simulink library "wabha_method"  (R2021b)
settings: Solver=VariableStepAuto  StartTime=0.0  StopTime=10.0  RelTol=1e-3
libraries: sharedutil x2, mat_3x3 x1
settings Model: Creator=white  LastModifiedBy=white

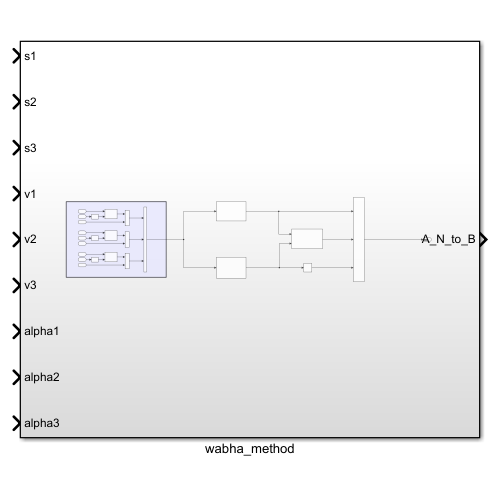
[thumbnail: Simulink's stored preview of the top-level diagram]
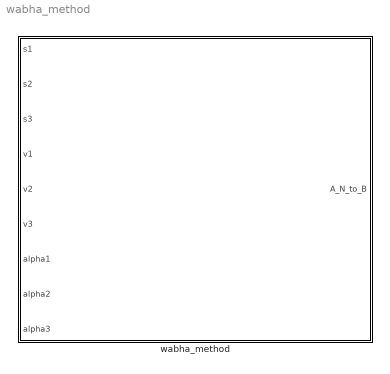
== system wabha_method ==
  wabha_method : Subsystem

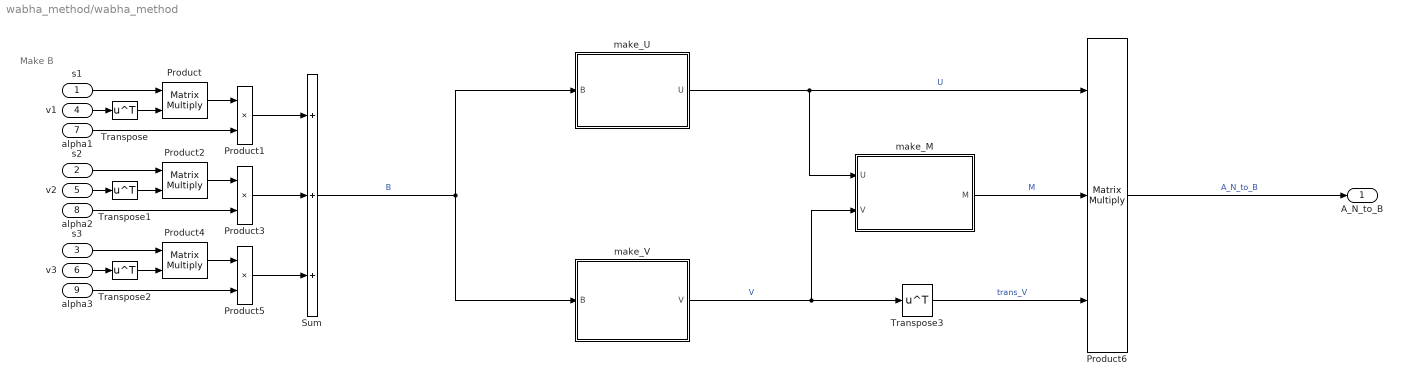
== system wabha_method/wabha_method ==
  note: Make B
  s1 : Inport
  s2 : Inport  Port=2
  s3 : Inport  Port=3
  v1 : Inport  Port=4
  v2 : Inport  Port=5
  v3 : Inport  Port=6
  alpha1 : Inport  Port=7
  alpha2 : Inport  Port=8
  alpha3 : Inport  Port=9
  Product : Product  Multiplication=Matrix(*)
  Product1 : Product
  Product2 : Product  Multiplication=Matrix(*)
  Product3 : Product
  Product4 : Product  Multiplication=Matrix(*)
  Product5 : Product
  Product6 : Product  Inputs=3  Multiplication=Matrix(*)
  Sum : Sum  Inputs=+++
  Transpose{,1..3} (4 alike) : Math  Operator=transpose  SaturateOnIntegerOverflow=on
  make_M : Subsystem
  make_U : Subsystem
  make_V : Subsystem
  A_N_to_B : Outport
  wires:
  v1/1 -> Transpose/1
  Transpose/1 -> Product/2
  s1/1 -> Product/1
  alpha1/1 -> Product1/2
  Product/1 -> Product1/1
  Product1/1 -> Sum/1
  Product2/1 -> Product3/1
  alpha2/1 -> Product3/2
  s2/1 -> Product2/1
  Transpose1/1 -> Product2/2
  v2/1 -> Transpose1/1
  Product3/1 -> Sum/2
  Product5/1 -> Sum/3
  v3/1 -> Transpose2/1
  Transpose2/1 -> Product4/2
  s3/1 -> Product4/1
  alpha3/1 -> Product5/2
  Product4/1 -> Product5/1
  Sum/1 -> make_V/1(B), make_U/1(B)  "B"
  make_U/1(U) -> make_M/1(U), Product6/1  "U"
  make_V/1(V) -> make_M/2(V), Transpose3/1  "V"
  Transpose3/1 -> Product6/3  "trans_V"
  make_M/1(M) -> Product6/2  "M"
  Product6/1 -> A_N_to_B/1  "A_N_to_B"

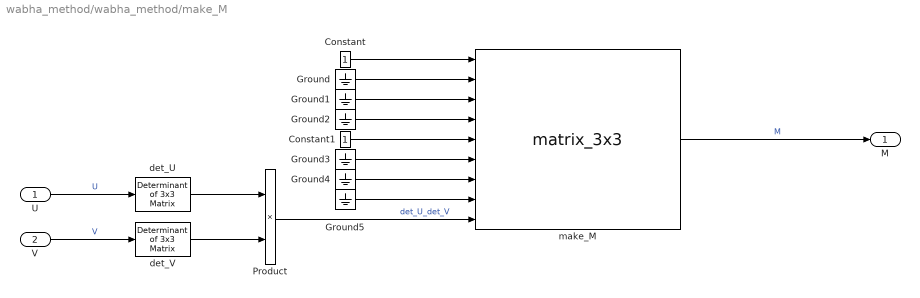
== system wabha_method/wabha_method/make_M ==
  U : Inport
  V : Inport  Port=2
  Constant : Constant
  Constant1 : Constant
  Ground{,1..5} (6 alike) : Ground
  Product : Product
  det_U : sharedutil/Determinant of 3x3 Matrix  aMode=aMode
      settings: SourceProductBaseCode=AE,PW,DR,MT,UV,VE
  det_V : sharedutil/Determinant of 3x3 Matrix  aMode=aMode
      settings: SourceProductBaseCode=AE,PW,DR,MT,UV,VE
  make_M : mat_3x3/matrix_3x3  SystemSampleTime=-1  VariantActivationTime=update diagram  Latency=0  AutoFrameSizeCalculation=off
  M : Outport
  wires:
  V/1 -> det_V/1  "V"
  U/1 -> det_U/1  "U"
  make_M/1 -> M/1  "M"
  Constant/1 -> make_M/1
  Ground/1 -> make_M/2
  Ground1/1 -> make_M/3
  Ground2/1 -> make_M/4
  Ground3/1 -> make_M/6
  Ground4/1 -> make_M/7
  Ground5/1 -> make_M/8
  Constant1/1 -> make_M/5
  det_V/1 -> Product/2
  det_U/1 -> Product/1
  Product/1 -> make_M/9  "det_U_det_V"

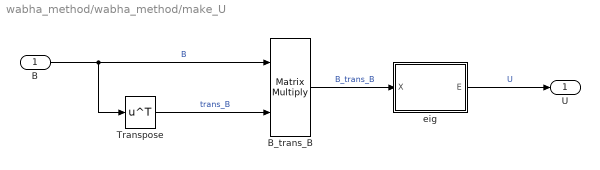
== system wabha_method/wabha_method/make_U ==
  B : Inport
  B_trans_B : Product  Multiplication=Matrix(*)
  Transpose : Math  Operator=transpose  SaturateOnIntegerOverflow=on
  eig : MATLAB Function  TreatAsAtomicUnit=on
  U : Outport
  wires:
  B/1 -> B_trans_B/1, Transpose/1  "B"
  Transpose/1 -> B_trans_B/2  "trans_B"
  B_trans_B/1 -> eig/1(X)  "B_trans_B"
  eig/1(E) -> U/1  "U"

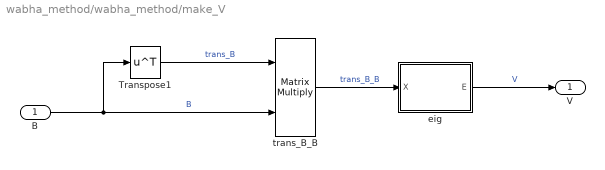
== system wabha_method/wabha_method/make_V ==
  B : Inport
  Transpose1 : Math  Operator=transpose  SaturateOnIntegerOverflow=on
  eig : MATLAB Function  TreatAsAtomicUnit=on
  trans_B_B : Product  Multiplication=Matrix(*)
  V : Outport
  wires:
  B/1 -> Transpose1/1, trans_B_B/2  "B"
  eig/1(E) -> V/1  "V"
  trans_B_B/1 -> eig/1(X)  "trans_B_B"
  Transpose1/1 -> trans_B_B/1  "trans_B"

== matlab function wabha_method/make_U/eig ==
  data: X input; E output
function E = eig_matrix(X)

[E, ~] = eig(X);

== matlab function wabha_method/make_V/eig ==
  data: X input; E output
function E = eig_matrix(X)

[E, ~] = eig(X);
